simulink model "steering_motor_smithPredictor"  (R2018b)
settings: Solver=VariableStepAuto  StartTime=0.0  StopTime=20  RelTol=1e-3
values from neighbouring files (symbols this model uses):
  D_steering_position = 0.0    (= 0)    [configuration.m]
  delay_tf_steering = 0    [configuration.m]
  den_tf_steering = [1 245.9 0]    [configuration.m]
  den_tf_steering_dis = [den_tf_steering_dis 0] - [0 den_tf_steering_dis]    [configuration.m]
  I_steering_position = 1    [configuration.m]    (also in simulate_bike.m = 30)
  initial_states = [deg2rad(-2) deg2rad(0) deg2rad(0)]    [configuration.m]    (also in configuration_pidTuning.m)
  num_tf_steering = [253.4]    [configuration.m]
  num_tf_steering_dis = [num_tf_steering_dis 0]    [configuration.m]
  P_steering_position = 10    [configuration.m]    (also in simulate_bike.m = 30)
  Ts = 0.01    [configuration.m]    (also in configuration_pidTuning.m = 0.04)
libraries: simulink x3
settings Model: Creator=maximef  LastModifiedBy=maximef

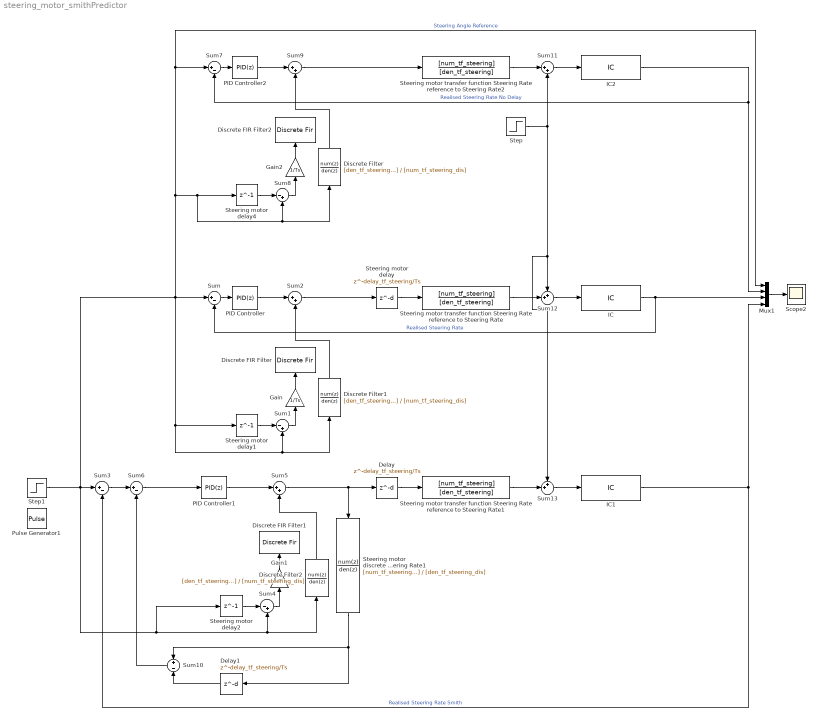
== system steering_motor_smithPredictor ==
  Delay : Delay  DelayLength=delay_tf_steering/Ts  SampleTime=Ts
  Delay1 : Delay  DelayLength=delay_tf_steering/Ts  SampleTime=Ts
  Discrete FIR Filter : DiscreteFir  SampleTime=Ts
  Discrete FIR Filter1 : DiscreteFir  SampleTime=Ts
  Discrete FIR Filter2 : DiscreteFir  SampleTime=Ts
  Discrete Filter : DiscreteFilter  Numerator=[den_tf_steering_dis]  Denominator=[num_tf_steering_dis]
  Discrete Filter1 : DiscreteFilter  Numerator=[den_tf_steering_dis]  Denominator=[num_tf_steering_dis]
  Discrete Filter2 : DiscreteFilter  Numerator=[den_tf_steering_dis]  Denominator=[num_tf_steering_dis]
  Gain : Gain  Gain=1/Ts
  Gain1 : Gain  Gain=1/Ts
  Gain2 : Gain  Gain=1/Ts
  IC : InitialCondition  Value=initial_states(2)
  IC1 : InitialCondition  Value=initial_states(2)
  IC2 : InitialCondition  Value=initial_states(2)
  Mux1 : Mux
  PID Controller : simulink/Continuous/PID Controller  Controller=PID  Form=Parallel  TimeDomain=Discrete-time  SampleTime=Ts  IntegratorMethod=Forward Euler  FilterMethod=Forward Euler  ControllerParametersSource=internal  P=P_steering_position  I=I_steering_position  D=D_steering_position  UseFilter=off  N=100  TunerSelectOption=Transfer Function Based (PID Tuner App)  InitialConditionSource=internal  InitialConditionForIntegrator=0  InitialConditionForFilter=0  DifferentiatorICPrevScaledInput=0  ExternalReset=none  TrackingMode=off  Kt=1  LimitOutput=off  UpperSaturationLimit=inf  LowerSaturationLimit=-inf  LinearizeAsGain=on  AntiWindupMode=none  Kb=1  POutMin=[]  POutMax=[]  IOutMin=[]  IOutMax=[]  DOutMin=[]  DOutMax=[]  NOutMin=[]  NOutMax=[]  SumOutMin=[]  SumOutMax=[]  SaturationOutMin=[]  SaturationOutMax=[]  PParamMin=[]  PParamMax=[]  IParamMin=[]  IParamMax=[]  DParamMin=[]  DParamMax=[]  NParamMin=[]  NParamMax=[]  KbParamMin=[]  KbParamMax=[]  KtParamMin=[]  KtParamMax=[]  KbOutMin=[]  KbOutMax=[]  KtOutMin=[]  KtOutMax=[]  IntegratorOutMin=[]  IntegratorOutMax=[]  FilterOutMin=[]  FilterOutMax=[]  SumI1OutMin=[]  SumI1OutMax=[]  SumI2OutMin=[]  SumI2OutMax=[]  SumI3OutMin=[]  SumI3OutMax=[]  SumI4OutMin=[]  SumI4OutMax=[]  SumDOutMin=[]  SumDOutMax=[]  DifferentiatorOutMin=[]  DifferentiatorOutMax=[]  FilterDiffOutCoefMin=[]  FilterDiffOutCoefMax=[]  ReciprocalOutMin=[]  ReciprocalOutMax=[]  SumDenOutMin=[]  SumDenOutMax=[]  SumNumOutMin=[]  SumNumOutMax=[]  DivideOutMin=[]  DivideOutMax=[]  IntegratorContinuousStateAttributes=''  IntegratorStateMustResolveToSignalObject=off  IntegratorRTWStateStorageClass=Auto  FilterContinuousStateAttributes=''  FilterStateMustResolveToSignalObject=off  FilterRTWStateStorageClass=Auto  ParallelPVariant=InternalParameters  IdealPVariant=Disabled  IVariant=InternalParameters  DVariant=InternalParameters  IntegratorVariant=Discrete  SatVariant=Disabled  AWVariant=Passthrough  PCopyVariant=Disabled  TRVariant=Disabled  FdbkBlocksVariant=Forward  IdealPFdbkVariant=Disabled  SatFdbkVariant=Disabled  DerivativeFilterVariant=Differentiator  NVariant=Passthrough  NCopyVariant=Disabled_SignalSpec  FilterICVariant=InternalICsDifferentiator  IntegratorICVariant=InternalICs  ExternalResetVariant=Disabled  TRSumVariant=Passthrough  SumFdbkVariant=Disabled  SumVariant=Sum_PID
  PID Controller1 : simulink/Continuous/PID Controller  Controller=PID  Form=Parallel  TimeDomain=Discrete-time  SampleTime=Ts  IntegratorMethod=Forward Euler  FilterMethod=Forward Euler  ControllerParametersSource=internal  P=P_steering_position  I=I_steering_position  D=D_steering_position  UseFilter=off  N=1  TunerSelectOption=Transfer Function Based (PID Tuner App)  InitialConditionSource=internal  InitialConditionForIntegrator=0  InitialConditionForFilter=0  DifferentiatorICPrevScaledInput=0  ExternalReset=none  TrackingMode=off  Kt=1  LimitOutput=off  UpperSaturationLimit=inf  LowerSaturationLimit=-inf  LinearizeAsGain=on  AntiWindupMode=none  Kb=1  POutMin=[]  POutMax=[]  IOutMin=[]  IOutMax=[]  DOutMin=[]  DOutMax=[]  NOutMin=[]  NOutMax=[]  SumOutMin=[]  SumOutMax=[]  SaturationOutMin=[]  SaturationOutMax=[]  PParamMin=[]  PParamMax=[]  IParamMin=[]  IParamMax=[]  DParamMin=[]  DParamMax=[]  NParamMin=[]  NParamMax=[]  KbParamMin=[]  KbParamMax=[]  KtParamMin=[]  KtParamMax=[]  KbOutMin=[]  KbOutMax=[]  KtOutMin=[]  KtOutMax=[]  IntegratorOutMin=[]  IntegratorOutMax=[]  FilterOutMin=[]  FilterOutMax=[]  SumI1OutMin=[]  SumI1OutMax=[]  SumI2OutMin=[]  SumI2OutMax=[]  SumI3OutMin=[]  SumI3OutMax=[]  SumI4OutMin=[]  SumI4OutMax=[]  SumDOutMin=[]  SumDOutMax=[]  DifferentiatorOutMin=[]  DifferentiatorOutMax=[]  FilterDiffOutCoefMin=[]  FilterDiffOutCoefMax=[]  ReciprocalOutMin=[]  ReciprocalOutMax=[]  SumDenOutMin=[]  SumDenOutMax=[]  SumNumOutMin=[]  SumNumOutMax=[]  DivideOutMin=[]  DivideOutMax=[]  IntegratorContinuousStateAttributes=''  IntegratorStateMustResolveToSignalObject=off  IntegratorRTWStateStorageClass=Auto  FilterContinuousStateAttributes=''  FilterStateMustResolveToSignalObject=off  FilterRTWStateStorageClass=Auto  ParallelPVariant=InternalParameters  IdealPVariant=Disabled  IVariant=InternalParameters  DVariant=InternalParameters  IntegratorVariant=Discrete  SatVariant=Disabled  AWVariant=Passthrough  PCopyVariant=Disabled  TRVariant=Disabled  FdbkBlocksVariant=Forward  IdealPFdbkVariant=Disabled  SatFdbkVariant=Disabled  DerivativeFilterVariant=Differentiator  NVariant=Passthrough  NCopyVariant=Disabled_SignalSpec  FilterICVariant=InternalICsDifferentiator  IntegratorICVariant=InternalICs  ExternalResetVariant=Disabled  TRSumVariant=Passthrough  SumFdbkVariant=Disabled  SumVariant=Sum_PID
  PID Controller2 : simulink/Continuous/PID Controller  Controller=PID  Form=Parallel  TimeDomain=Discrete-time  SampleTime=Ts  IntegratorMethod=Forward Euler  FilterMethod=Forward Euler  ControllerParametersSource=internal  P=P_steering_position  I=I_steering_position  D=D_steering_position  UseFilter=off  N=100  TunerSelectOption=Transfer Function Based (PID Tuner App)  InitialConditionSource=internal  InitialConditionForIntegrator=0  InitialConditionForFilter=0  DifferentiatorICPrevScaledInput=0  ExternalReset=none  TrackingMode=off  Kt=1  LimitOutput=off  UpperSaturationLimit=inf  LowerSaturationLimit=-inf  LinearizeAsGain=on  AntiWindupMode=none  Kb=1  POutMin=[]  POutMax=[]  IOutMin=[]  IOutMax=[]  DOutMin=[]  DOutMax=[]  NOutMin=[]  NOutMax=[]  SumOutMin=[]  SumOutMax=[]  SaturationOutMin=[]  SaturationOutMax=[]  PParamMin=[]  PParamMax=[]  IParamMin=[]  IParamMax=[]  DParamMin=[]  DParamMax=[]  NParamMin=[]  NParamMax=[]  KbParamMin=[]  KbParamMax=[]  KtParamMin=[]  KtParamMax=[]  KbOutMin=[]  KbOutMax=[]  KtOutMin=[]  KtOutMax=[]  IntegratorOutMin=[]  IntegratorOutMax=[]  FilterOutMin=[]  FilterOutMax=[]  SumI1OutMin=[]  SumI1OutMax=[]  SumI2OutMin=[]  SumI2OutMax=[]  SumI3OutMin=[]  SumI3OutMax=[]  SumI4OutMin=[]  SumI4OutMax=[]  SumDOutMin=[]  SumDOutMax=[]  DifferentiatorOutMin=[]  DifferentiatorOutMax=[]  FilterDiffOutCoefMin=[]  FilterDiffOutCoefMax=[]  ReciprocalOutMin=[]  ReciprocalOutMax=[]  SumDenOutMin=[]  SumDenOutMax=[]  SumNumOutMin=[]  SumNumOutMax=[]  DivideOutMin=[]  DivideOutMax=[]  IntegratorContinuousStateAttributes=''  IntegratorStateMustResolveToSignalObject=off  IntegratorRTWStateStorageClass=Auto  FilterContinuousStateAttributes=''  FilterStateMustResolveToSignalObject=off  FilterRTWStateStorageClass=Auto  ParallelPVariant=InternalParameters  IdealPVariant=Disabled  IVariant=InternalParameters  DVariant=InternalParameters  IntegratorVariant=Discrete  SatVariant=Disabled  AWVariant=Passthrough  PCopyVariant=Disabled  TRVariant=Disabled  FdbkBlocksVariant=Forward  IdealPFdbkVariant=Disabled  SatFdbkVariant=Disabled  DerivativeFilterVariant=Differentiator  NVariant=Passthrough  NCopyVariant=Disabled_SignalSpec  FilterICVariant=InternalICsDifferentiator  IntegratorICVariant=InternalICs  ExternalResetVariant=Disabled  TRSumVariant=Passthrough  SumFdbkVariant=Disabled  SumVariant=Sum_PID
  Pulse Generator1 : DiscretePulseGenerator  PulseType=Time based  Amplitude=deg2rad(10)  Period=5  PulseWidth=50
  Scope2 : Scope
  Steering motor delay : Delay  DelayLength=delay_tf_steering/Ts  SampleTime=Ts
  Steering motor delay1 : Delay  DelayLength=1  SampleTime=Ts
  Steering motor delay2 : Delay  DelayLength=1  SampleTime=Ts
  Steering motor delay4 : Delay  DelayLength=1  SampleTime=Ts
  Steering motor discrete transfer function Steering Rate reference to Steering Rate1 : DiscreteTransferFcn  Numerator=[num_tf_steering_dis]  Denominator=[den_tf_steering_dis]  SampleTime=Ts
  Steering motor transfer function Steering Rate reference to Steering Rate : TransferFcn  Numerator=[num_tf_steering]  Denominator=[den_tf_steering]
  Steering motor transfer function Steering Rate reference to Steering Rate1 : TransferFcn  Numerator=[num_tf_steering]  Denominator=[den_tf_steering]
  Steering motor transfer function Steering Rate reference to Steering Rate2 : TransferFcn  Numerator=[num_tf_steering]  Denominator=[den_tf_steering]
  Step : Step  Time=10  After=deg2rad(3)  SampleTime=0
  Step1 : Step  After=deg2rad(10)  SampleTime=Ts
  Sum{,3,6..7} (4 alike) : Sum  Inputs=|+-
  Sum1 : Sum  Inputs=|-+
  Sum10 : Sum  Inputs=+-
  Sum{2,5,9,11} (4 alike) : Sum  Inputs=|++
  Sum12 : Sum  Inputs=++|
  Sum13 : Sum  Inputs=++|
  Sum4 : Sum  Inputs=|-+
  Sum8 : Sum  Inputs=|-+
  wires:
  Steering motor delay/1 -> Steering motor transfer function Steering Rate reference to Steering Rate/1
  PID Controller/1 -> Sum2/1
  Sum/1 -> PID Controller/1
  Steering motor delay1/1 -> Sum1/1
  Sum2/1 -> Steering motor delay/1
  Sum1/1 -> Gain/1
  Gain/1 -> Discrete FIR Filter/1
  Sum10/1 -> Sum6/2
  Steering motor discrete transfer function Steering Rate reference to Steering Rate1/1 -> Sum10/1, Delay1/1
  Sum3/1 -> Sum6/1
  Sum4/1 -> Gain1/1
  Gain1/1 -> Discrete FIR Filter1/1
  Mux1/1 -> Scope2/1
  PID Controller1/1 -> Sum5/1
  Sum5/1 -> Delay/1, Steering motor discrete transfer function Steering Rate reference to Steering Rate1/1
  Steering motor delay2/1 -> Sum4/1
  Delay/1 -> Steering motor transfer function Steering Rate reference to Steering Rate1/1
  Steering motor transfer function Steering Rate reference to Steering Rate1/1 -> Sum13/2
  IC/1 -> Mux1/3, Sum/2  "Realised Steering Rate"
  IC1/1 -> Sum3/2, Mux1/4  "Realised Steering Rate Smith"
  Sum11/1 -> IC2/1
  IC2/1 -> Sum7/2, Mux1/2  "Realised Steering Rate No Delay"
  Steering motor delay4/1 -> Sum8/1
  Sum7/1 -> PID Controller2/1
  Sum8/1 -> Gain2/1
  Step1/1 -> Sum7/1, Mux1/1, Steering motor delay4/1, Discrete Filter/1, Sum8/2, Discrete Filter1/1, Sum1/2, Steering motor delay1/1, Sum/1, Steering motor delay2/1, Discrete Filter2/1, Sum4/2, Sum3/1  "Steering Angle Reference"
  PID Controller2/1 -> Sum9/1
  Gain2/1 -> Discrete FIR Filter2/1
  Sum9/1 -> Steering motor transfer function Steering Rate reference to Steering Rate2/1
  Delay1/1 -> Sum10/2
  Discrete Filter/1 -> Sum9/2
  Discrete Filter1/1 -> Sum2/2
  Discrete Filter2/1 -> Sum5/2
  Sum6/1 -> PID Controller1/1
  Step/1 -> Sum13/1, Sum12/1, Sum11/2
  Steering motor transfer function Steering Rate reference to Steering Rate2/1 -> Sum11/1
  Sum12/1 -> IC/1
  Steering motor transfer function Steering Rate reference to Steering Rate/1 -> Sum12/2
  Sum13/1 -> IC1/1
